simulink model "eps_fix"  (R2019b)
settings: Solver=VariableStepAuto  StartTime=0.0  StopTime=10.0  RelTol=1e-3
values from neighbouring files (symbols this model uses):
  Moment_limit = reshape([momen{:}],size(momen))    [Lookup_table.m]
  Steering_Angle = reshape([angle{:}],size(angle))    [Lookup_table.m]
  Vehicle_Speed = reshape([speed{:}],size(speed))    [Lookup_table.m]
undefined symbols (not defined in the file or in its folder): Moment_limit_am, Steering_Angle_am
libraries: simulink x1
settings Model: Creator=DUY  LastModifiedBy=DUY

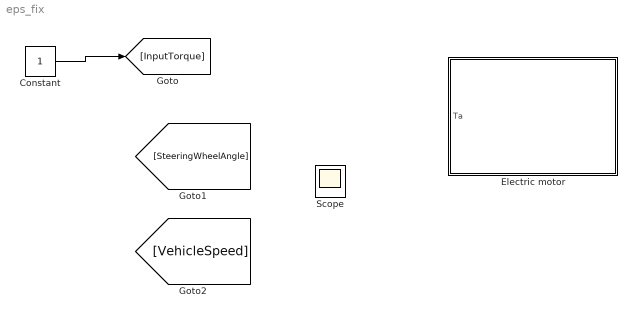
== system eps_fix ==
  Constant : Constant
  Electric motor : Subsystem
      mask Display: image('D:\MATLAB Projects\MATLAB_EPS_Complete_09_05\CapsoneProject\duy\mask\5dm33752-mechatronika-eps_eda_text-image_textimage.jpg'); % Use "Edit Image" on toolstrip to change.
  Scope : Scope
  wires:
  Constant/1 -> [InputTorque]

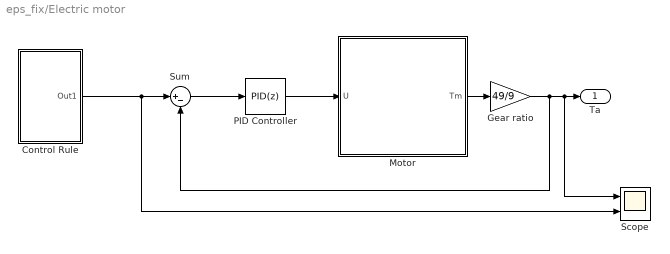
== system eps_fix/Electric motor ==
  Control Rule : Subsystem
  Gear ratio : Gain  Gain=49/9
  "Motor " : Subsystem  mask{Km=0.456, Kb=0.3533, B=0.071, J=0.00218907, L=0.002, R=0.6}
      mask prompts: Km "Torque constant"; Kb "Back emf constant"; B "Viscous friction"; J "Inertia"; L "Inductance"; R "Resistance"
      mask Display: image('motor.png');
  PID Controller : simulink/Continuous/PID Controller  Controller=PID  Form=Parallel  TimeDomain=Discrete-time  SampleTime=-1  IntegratorMethod=Forward Euler  FilterMethod=Forward Euler  ControllerParametersSource=internal  P=0.45  I=128  D=100  UseFilter=off  N=0  TunerSelectOption=Transfer Function Based (PID Tuner App)  InitialConditionSource=internal  InitialConditionForIntegrator=0  InitialConditionForFilter=0  DifferentiatorICPrevScaledInput=0  ExternalReset=none  TrackingMode=off  Kt=1  LimitOutput=on  UpperSaturationLimit=36  LowerSaturationLimit=-36  LinearizeAsGain=on  AntiWindupMode=none  Kb=1  POutMin=[]  POutMax=[]  IOutMin=[]  IOutMax=[]  DOutMin=[]  DOutMax=[]  NOutMin=[]  NOutMax=[]  SumOutMin=[]  SumOutMax=[]  SaturationOutMin=[]  SaturationOutMax=[]  PParamMin=[]  PParamMax=[]  IParamMin=[]  IParamMax=[]  DParamMin=[]  DParamMax=[]  NParamMin=[]  NParamMax=[]  KbParamMin=[]  KbParamMax=[]  KtParamMin=[]  KtParamMax=[]  KbOutMin=[]  KbOutMax=[]  KtOutMin=[]  KtOutMax=[]  IntegratorOutMin=[]  IntegratorOutMax=[]  FilterOutMin=[]  FilterOutMax=[]  SumI1OutMin=[]  SumI1OutMax=[]  SumI2OutMin=[]  SumI2OutMax=[]  SumI3OutMin=[]  SumI3OutMax=[]  SumI4OutMin=[]  SumI4OutMax=[]  SumDOutMin=[]  SumDOutMax=[]  DifferentiatorOutMin=[]  DifferentiatorOutMax=[]  FilterDiffOutCoefMin=[]  FilterDiffOutCoefMax=[]  ReciprocalOutMin=[]  ReciprocalOutMax=[]  SumDenOutMin=[]  SumDenOutMax=[]  SumNumOutMin=[]  SumNumOutMax=[]  DivideOutMin=[]  DivideOutMax=[]  IntegratorContinuousStateAttributes=''  IntegratorStateMustResolveToSignalObject=off  IntegratorRTWStateStorageClass=Auto  FilterContinuousStateAttributes=''  FilterStateMustResolveToSignalObject=off  FilterRTWStateStorageClass=Auto  ParallelPVariant=InternalParameters  IdealPVariant=Disabled  IVariant=InternalParameters  DVariant=InternalParameters  IntegratorVariant=Discrete  SatVariant=Enabled  AWVariant=Passthrough  PCopyVariant=Disabled  TRVariant=Disabled  FdbkBlocksVariant=Forward  IdealPFdbkVariant=Disabled  SatFdbkVariant=Disabled  DerivativeFilterVariant=Differentiator  NVariant=Passthrough  NCopyVariant=Disabled_SignalSpec  FilterICVariant=InternalICsDifferentiator  IntegratorICVariant=InternalICs  ExternalResetVariant=Disabled  TRSumVariant=Passthrough  SumFdbkVariant=Disabled  SumVariant=Sum_PID
  Scope : Scope  NumInputPorts=2
  Sum : Sum  Inputs=|+-
  Ta : Outport
  wires:
  PID Controller/1 -> "Motor "/1(U)
  "Motor "/1(Tm) -> Gear ratio/1
  Sum/1 -> PID Controller/1
  Control Rule/1(Out1) -> Scope/2, Sum/1
  Gear ratio/1 -> Sum/2, Scope/1, Ta/1

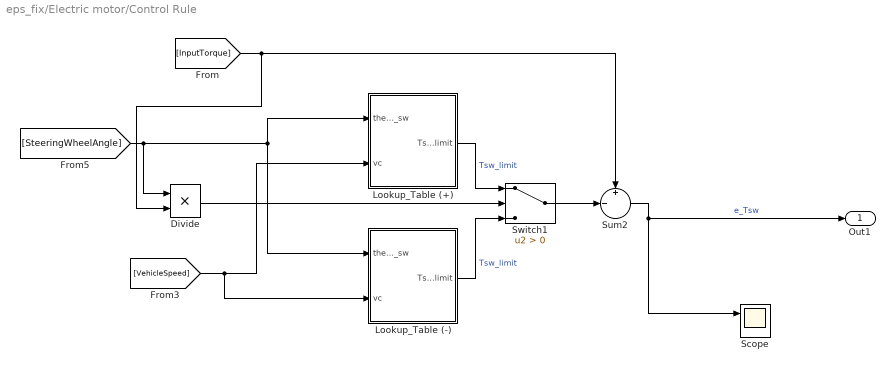
== system eps_fix/Electric motor/Control Rule ==
  Divide : Product  Inputs=**
  Lookup_Table (+) : Subsystem
  Lookup_Table (-) : Subsystem
  Scope : Scope  NumInputPorts=2
  Sum2 : Sum  Inputs=+|-||
  Switch1 : Switch  Criteria=u2 > Threshold
  Out1 : Outport
  wires:
  [InputTorque] -> Divide/2, Sum2/1
  Sum2/1 -> Out1/1, Scope/1  "e_Tsw"
  [VehicleSpeed] -> Lookup_Table (-)/2(vc), Lookup_Table (+)/2(vc)
  Lookup_Table (+)/1(Tsw_limit) -> Switch1/1  "Tsw_limit"
  Lookup_Table (-)/1(Tsw_limit) -> Switch1/3  "Tsw_limit"
  [SteeringWheelAngle] -> Divide/1, Lookup_Table (-)/1(theta_sw), Lookup_Table (+)/1(theta_sw)
  Switch1/1 -> Sum2/2
  Divide/1 -> Switch1/2

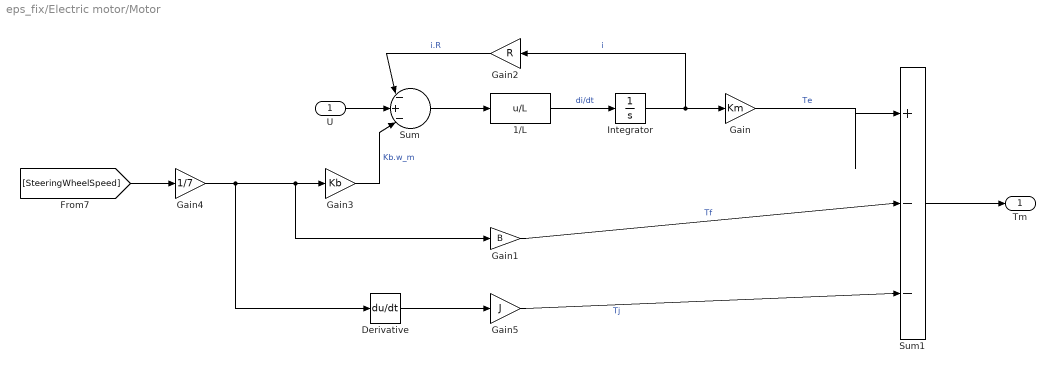
== system eps_fix/Electric motor/Motor  ==
  U : Inport
  1/L : Fcn  Expr=u/L
  Derivative : Derivative
  Gain : Gain  Gain=Km
  Gain1 : Gain  Gain=B
  Gain2 : Gain  Gain=R
  Gain3 : Gain  Gain=Kb
  Gain4 : Gain  Gain=1/7
  Gain5 : Gain  Gain=J
  Integrator : Integrator
  Sum : Sum  Inputs=|-+-|
  Sum1 : Sum  Inputs=|+--
  Tm : Outport  VectorParamsAs1DForOutWhenUnconnected=off
  wires:
  Sum/1 -> 1/L/1
  1/L/1 -> Integrator/1  "di/dt"
  Integrator/1 -> Gain2/1, Gain/1  "i"
  Gain/1 -> Sum1/1  "Te"
  Gain2/1 -> Sum/1  "i.R"
  Gain1/1 -> Sum1/2  "Tf"
  Sum1/1 -> Tm/1
  Derivative/1 -> Gain5/1
  Gain5/1 -> Sum1/3  "Tj"
  [SteeringWheelSpeed] -> Gain4/1
  U/1 -> Sum/2
  Gain3/1 -> Sum/3  "Kb.w_m"
  Gain4/1 -> Derivative/1, Gain1/1, Gain3/1

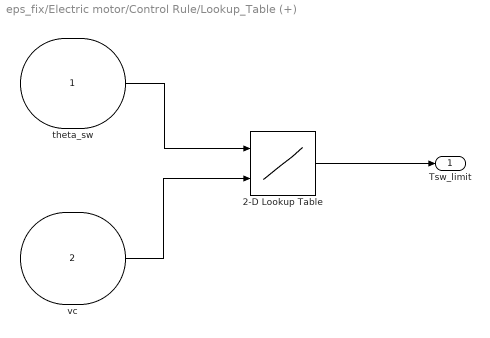
== system eps_fix/Electric motor/Control Rule/Lookup_Table (+) ==
  theta_sw : Inport
      mask Display: image('1.png');
  vc : Inport  Port=2
      mask Display: image('speed.png');
  2-D Lookup Table : Lookup_n-D  BreakpointsForDimension1=Steering_Angle  BreakpointsForDimension2=Vehicle_Speed  Table=Moment_limit  InternalRulePriority=Speed  RndMeth=Simplest  InputSameDT=on
  Tsw_limit : Outport  VectorParamsAs1DForOutWhenUnconnected=off
  wires:
  theta_sw/1 -> 2-D Lookup Table/1
  vc/1 -> 2-D Lookup Table/2
  2-D Lookup Table/1 -> Tsw_limit/1

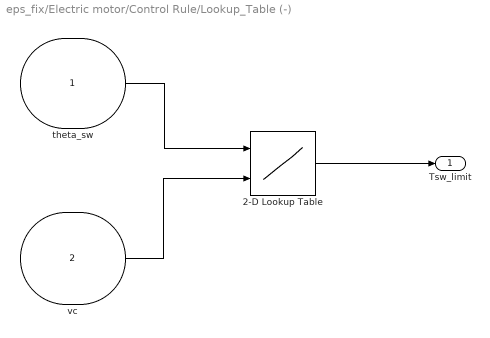
== system eps_fix/Electric motor/Control Rule/Lookup_Table (-) ==
  theta_sw : Inport
      mask Display: image('1.png');
  vc : Inport  Port=2
      mask Display: image('speed.png');
  2-D Lookup Table : Lookup_n-D  BreakpointsForDimension1=Steering_Angle_am  BreakpointsForDimension2=Vehicle_Speed  Table=Moment_limit_am  InternalRulePriority=Speed  RndMeth=Simplest  InputSameDT=on
  Tsw_limit : Outport  VectorParamsAs1DForOutWhenUnconnected=off
  wires:
  2-D Lookup Table/1 -> Tsw_limit/1
  vc/1 -> 2-D Lookup Table/2
  theta_sw/1 -> 2-D Lookup Table/1
